simulink model "T37_v65_2015b"  (Simulink 8.6)
settings: Solver=ode45  StartTime=0.0  StopTime=180  FixedStep=0.001  MaxStep=0.1  RelTol=1e-3
values from neighbouring files (symbols this model uses):
  Aero_RP = Aero_RP*[-1 0 0;0 1 0;0 0 -1]    [t37_data.m]
  aileron_limits = [-0.35 0.35]*pi/180    [t37_data.m]
  CD_alpha = 0.3840    (= 0.384)    [t37_data.m]
  CD_beta = [-1.5700	1.2300 ... (first row only)    [t37_data.m]
  CD_flap = 0.0750    (= 0.075)    [t37_data.m]
  CD_zero = [  -1.5700	1.5000 ... (first row only)    [t37_data.m]
  Cl_ail = [0.0000	0.1810 ... (first row only)    [t37_data.m]
  CL_alpha = [-0.2000	-0.6400 ... (first row only)    [t37_data.m]
  CL_alpha_dot = 2.0    (= 2)    [t37_data.m]
  Cl_beta = -0.0944    [t37_data.m]
  CL_elev = 0.5    [t37_data.m]
  CL_flap = 0.3500    (= 0.35)    [t37_data.m]
  CL_ground_effect = [0.0000	1.0610 ... (first row only)    [t37_data.m]
  Cl_p = -0.4420    (= -0.442)    [t37_data.m]
  CL_q = 4.1    [t37_data.m]
  Cl_r = 0.0926    [t37_data.m]
  Cl_rudder = 0.0150    (= 0.015)    [t37_data.m]
  Cm_alpha = -0.7000    (= -0.7)    [t37_data.m]
  Cm_alpha_dot = -6.9500    (= -6.95)    [t37_data.m]
  Cm_elev = [0.0000	-1.1200 ... (first row only)    [t37_data.m]
  Cm_q = -50.0000    (= -50)    [t37_data.m]
  Cm_zero = 0.0250    (= 0.025)    [t37_data.m]
  Cn_beta = 0.1106    [t37_data.m]
  Cn_p = -0.0243    [t37_data.m]
  Cn_r = -0.1390    (= -0.139)    [t37_data.m]
  Cn_rudder = -0.0365    [t37_data.m]
  CY_beta = -0.3460    (= -0.346)    [t37_data.m]
  CY_p = -0.0827    [t37_data.m]
  CY_r = 0.3000    (= 0.3)    [t37_data.m]
  CY_rudder = 0.200    (= 0.2)    [t37_data.m]
  elevator_limits = [-0.35 0.3]*pi/180    [t37_data.m]
  isTrimming = 0    [mytrim.m]    (also in t37_data.m)
  Jxx = 7985*1.3558179    (= 10826.2059315)    [t37_data.m]
  Jxz = 0    [t37_data.m]
  Jyy = 6000*1.3558179    (= 8134.9074)    [t37_data.m]
  Jzz = 11183*1.3558179    (= 15162.1115757)    [t37_data.m]
  M = 4056*0.45359237    (= 1839.77065272)    [t37_data.m]
  Rcg = Rcg*[-1 0 0;0 1 0;0 0 -1]    [t37_data.m]
  Rengine1 = Rengine1*[-1 0 0;0 1 0;0 0 -1]    [t37_data.m]
  Rengine2 = Rengine2*[-1 0 0;0 1 0;0 0 -1]    [t37_data.m]
  rudder_limits = [-0.35 0.35]*pi/180    [t37_data.m]
  Sw = 182*0.09290304    (= 16.90835328)    [t37_data.m]
  thrust_limits = [0 1]    [t37_data.m]
  Tmax = M*10    (= 18397.7065272)    [t37_data.m]
  u0 = [ ... (first row only)    [mytrim.m]    (also in t37_data.m = zeros(4,1))
  x0 = [ ... (first row only)    [mytrim.m]    (also in t37_data.m = zeros(12,1))
undefined symbols (not defined in the file or in its folder): CD_elevator
undefined symbols (not defined in the file): Bw, Cw
(part 2 of 2)

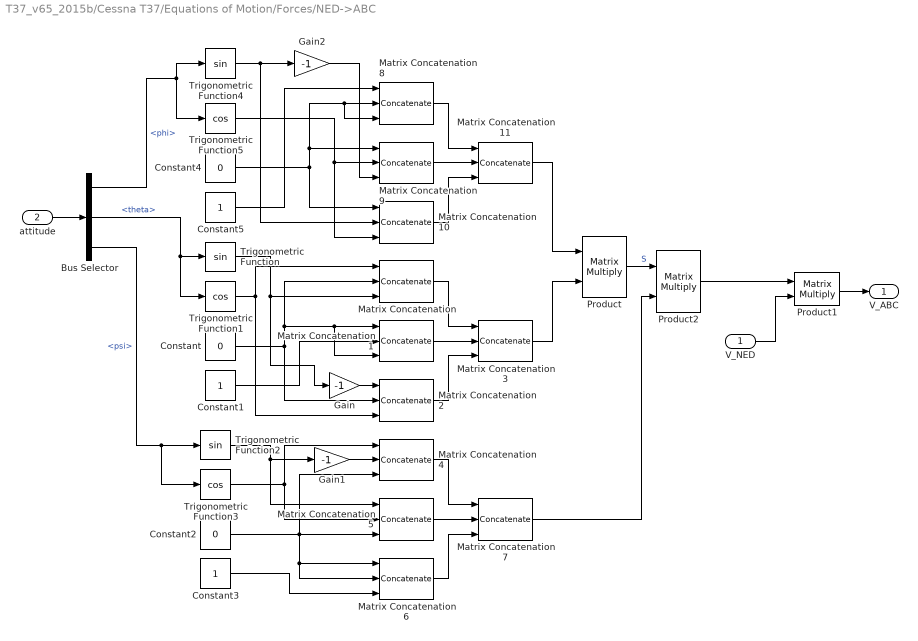
== system T37_v65_2015b/Cessna T37/Equations of Motion/Forces/NED->ABC ==
  V_NED : Inport
  attitude : Inport  Port=2
  Bus Selector : BusSelector  OutputSignals=phi,theta,psi
  Constant : Constant  Value=0
  Constant1 : Constant
  Constant2 : Constant  Value=0
  Constant3 : Constant
  Constant4 : Constant  Value=0
  Constant5 : Constant
  Gain : Gain  Gain=-1  SaturateOnIntegerOverflow=on  OutDataTypeStr=Inherit: Same as input  ParamDataTypeStr=Inherit: Same as input
  Gain1 : Gain  Gain=-1  SaturateOnIntegerOverflow=on  OutDataTypeStr=Inherit: Same as input  ParamDataTypeStr=Inherit: Same as input
  Gain2 : Gain  Gain=-1  SaturateOnIntegerOverflow=on  OutDataTypeStr=Inherit: Same as input  ParamDataTypeStr=Inherit: Same as input
  Matrix Concatenation{,1..2,4..6,8..10} (9 alike) : Concatenate  NumInputs=3  Mode=Multidimensional array
  Matrix Concatenation11 : Concatenate  NumInputs=3  Mode=Multidimensional array  ConcatenateDimension=2
  Matrix Concatenation3 : Concatenate  NumInputs=3  Mode=Multidimensional array  ConcatenateDimension=2
  Matrix Concatenation7 : Concatenate  NumInputs=3  Mode=Multidimensional array  ConcatenateDimension=2
  Product : Product  Multiplication=Matrix(*)  SaturateOnIntegerOverflow=on  OutDataTypeStr=Inherit: Same as first input
  Product1 : Product  Multiplication=Matrix(*)  SaturateOnIntegerOverflow=on  OutDataTypeStr=Inherit: Same as first input
  Product2 : Product  Multiplication=Matrix(*)  SaturateOnIntegerOverflow=on  OutDataTypeStr=Inherit: Same as first input
  Trigonometric Function : Trigonometry
  Trigonometric Function1 : Trigonometry  Operator=cos
  Trigonometric Function2 : Trigonometry
  Trigonometric Function3 : Trigonometry  Operator=cos
  Trigonometric Function4 : Trigonometry
  Trigonometric Function5 : Trigonometry  Operator=cos
  V_ABC : Outport
  wires:
  Trigonometric Function1/1 -> Matrix Concatenation/1, Matrix Concatenation2/3
  Trigonometric Function/1 -> Matrix Concatenation/3, Gain/1
  Constant/1 -> Matrix Concatenation/2, Matrix Concatenation1/1, Matrix Concatenation1/3, Matrix Concatenation2/2
  Constant1/1 -> Matrix Concatenation1/2
  Matrix Concatenation/1 -> Matrix Concatenation3/1
  Matrix Concatenation1/1 -> Matrix Concatenation3/2
  Matrix Concatenation2/1 -> Matrix Concatenation3/3
  Matrix Concatenation4/1 -> Matrix Concatenation7/1
  Matrix Concatenation5/1 -> Matrix Concatenation7/2
  Matrix Concatenation6/1 -> Matrix Concatenation7/3
  Trigonometric Function3/1 -> Matrix Concatenation4/1, Matrix Concatenation5/2
  Trigonometric Function2/1 -> Gain1/1, Matrix Concatenation5/1
  Constant2/1 -> Matrix Concatenation4/3, Matrix Concatenation5/3, Matrix Concatenation6/1, Matrix Concatenation6/2
  Constant3/1 -> Matrix Concatenation6/3
  Product1/1 -> V_ABC/1
  attitude/1 -> Bus Selector/1
  Matrix Concatenation8/1 -> Matrix Concatenation11/1
  Matrix Concatenation9/1 -> Matrix Concatenation11/2
  Matrix Concatenation10/1 -> Matrix Concatenation11/3
  Bus Selector/1 -> Trigonometric Function4/1, Trigonometric Function5/1  "<phi>"
  Constant5/1 -> Matrix Concatenation8/1
  Constant4/1 -> Matrix Concatenation8/2, Matrix Concatenation8/3, Matrix Concatenation9/1, Matrix Concatenation10/1
  Trigonometric Function5/1 -> Matrix Concatenation9/2, Matrix Concatenation10/3
  Trigonometric Function4/1 -> Matrix Concatenation10/2, Gain2/1
  Bus Selector/2 -> Trigonometric Function/1, Trigonometric Function1/1  "<theta>"
  Bus Selector/3 -> Trigonometric Function2/1, Trigonometric Function3/1  "<psi>"
  Matrix Concatenation11/1 -> Product/1
  Matrix Concatenation3/1 -> Product/2
  V_NED/1 -> Product1/2
  Product/1 -> Product2/1  "S"
  Matrix Concatenation7/1 -> Product2/2
  Product2/1 -> Product1/1
  Gain2/1 -> Matrix Concatenation9/3
  Gain/1 -> Matrix Concatenation2/1
  Gain1/1 -> Matrix Concatenation4/2

== system T37_v65_2015b/Cessna T37/Equations of Motion/Forces/Produto Vetorial ==
  V1 : Inport
  V2 : Inport  Port=2
  Mux : Mux  Inputs=2
  Mux1 : Mux  Inputs=3
  i : Fcn  Expr=u(2)*u(6)-u(3)*u(5)
  j : Fcn  Expr=-u(1)*u(6)+u(3)*u(4)
  k : Fcn  Expr=u(1)*u(5)-u(2)*u(4)
  V1 x V2 : Outport
  wires:
  V1/1 -> Mux/1
  V2/1 -> Mux/2
  Mux/1 -> i/1, j/1, k/1
  i/1 -> Mux1/1
  j/1 -> Mux1/2
  k/1 -> Mux1/3
  Mux1/1 -> V1 x V2/1

== system T37_v65_2015b/Cessna T37/Equations of Motion/Forces/Produto Vetorial1 ==
  V1 : Inport
  V2 : Inport  Port=2
  Mux : Mux  Inputs=2
  Mux1 : Mux  Inputs=3
  i : Fcn  Expr=u(2)*u(6)-u(3)*u(5)
  j : Fcn  Expr=-u(1)*u(6)+u(3)*u(4)
  k : Fcn  Expr=u(1)*u(5)-u(2)*u(4)
  V1 x V2 : Outport
  wires:
  V1/1 -> Mux/1
  V2/1 -> Mux/2
  Mux/1 -> i/1, j/1, k/1
  i/1 -> Mux1/1
  j/1 -> Mux1/2
  k/1 -> Mux1/3
  Mux1/1 -> V1 x V2/1

== system T37_v65_2015b/Cessna T37/Equations of Motion/Forces/Produto Vetorial2 ==
  V1 : Inport
  V2 : Inport  Port=2
  Mux : Mux  Inputs=2
  Mux1 : Mux  Inputs=3
  i : Fcn  Expr=u(2)*u(6)-u(3)*u(5)
  j : Fcn  Expr=-u(1)*u(6)+u(3)*u(4)
  k : Fcn  Expr=u(1)*u(5)-u(2)*u(4)
  V1 x V2 : Outport
  wires:
  V1/1 -> Mux/1
  V2/1 -> Mux/2
  Mux/1 -> i/1, j/1, k/1
  i/1 -> Mux1/1
  j/1 -> Mux1/2
  k/1 -> Mux1/3
  Mux1/1 -> V1 x V2/1

== system T37_v65_2015b/Cessna T37/Equations of Motion/Forces/Produto Vetorial3 ==
  V1 : Inport
  V2 : Inport  Port=2
  Mux : Mux  Inputs=2
  Mux1 : Mux  Inputs=3
  i : Fcn  Expr=u(2)*u(6)-u(3)*u(5)
  j : Fcn  Expr=-u(1)*u(6)+u(3)*u(4)
  k : Fcn  Expr=u(1)*u(5)-u(2)*u(4)
  V1 x V2 : Outport
  wires:
  V1/1 -> Mux/1
  V2/1 -> Mux/2
  Mux/1 -> i/1, j/1, k/1
  i/1 -> Mux1/1
  j/1 -> Mux1/2
  k/1 -> Mux1/3
  Mux1/1 -> V1 x V2/1

== system T37_v65_2015b/Cessna T37/Equations of Motion/Moments/Inertia ==
  Constant : Constant  Value=Jxx
  Constant1 : Constant  Value=Jyy
  Constant2 : Constant  Value=Jzz
  Constant3 : Constant  Value=-Jxz
  Constant4 : Constant  Value=0
  Matrix Concatenation10 : Concatenate  NumInputs=3  Mode=Multidimensional array
  Matrix Concatenation11 : Concatenate  NumInputs=3  Mode=Multidimensional array  ConcatenateDimension=2
  Matrix Concatenation8 : Concatenate  NumInputs=3  Mode=Multidimensional array
  Matrix Concatenation9 : Concatenate  NumInputs=3  Mode=Multidimensional array
  J : Outport
  wires:
  Matrix Concatenation8/1 -> Matrix Concatenation11/1
  Matrix Concatenation9/1 -> Matrix Concatenation11/2
  Matrix Concatenation10/1 -> Matrix Concatenation11/3
  Matrix Concatenation11/1 -> J/1
  Constant/1 -> Matrix Concatenation8/1
  Constant4/1 -> Matrix Concatenation8/2, Matrix Concatenation9/1, Matrix Concatenation9/3, Matrix Concatenation10/2
  Constant3/1 -> Matrix Concatenation8/3, Matrix Concatenation10/1
  Constant1/1 -> Matrix Concatenation9/2
  Constant2/1 -> Matrix Concatenation10/3

== system T37_v65_2015b/Cessna T37/Equations of Motion/Moments/Inverse Inertia Matrix ==
  Constant : Constant  Value=Jzz
  Constant1 : Constant  Value=1/Jyy
  Constant2 : Constant  Value=Jxx
  Constant3 : Constant  Value=Jxz
  Constant4 : Constant  Value=0
  Constant5 : Constant  Value=Jxx*Jzz-Jxz^2
  Matrix Concatenation10 : Concatenate  NumInputs=3  Mode=Multidimensional array
  Matrix Concatenation11 : Concatenate  NumInputs=3  Mode=Multidimensional array  ConcatenateDimension=2
  Matrix Concatenation8 : Concatenate  NumInputs=3  Mode=Multidimensional array
  Matrix Concatenation9 : Concatenate  NumInputs=3  Mode=Multidimensional array
  Product : Product  Inputs=*/  SaturateOnIntegerOverflow=on  OutDataTypeStr=Inherit: Same as first input
  Product1 : Product  SaturateOnIntegerOverflow=on  OutDataTypeStr=Inherit: Same as first input
  inv J : Outport
  wires:
  Matrix Concatenation8/1 -> Matrix Concatenation11/1
  Matrix Concatenation9/1 -> Matrix Concatenation11/2
  Matrix Concatenation10/1 -> Matrix Concatenation11/3
  Constant/1 -> Matrix Concatenation8/1
  Constant4/1 -> Matrix Concatenation8/2, Matrix Concatenation9/1, Matrix Concatenation9/3, Matrix Concatenation10/2
  Constant3/1 -> Matrix Concatenation8/3, Matrix Concatenation10/1
  Constant2/1 -> Matrix Concatenation10/3
  Matrix Concatenation11/1 -> Product/1
  Product/1 -> inv J/1
  Constant5/1 -> Product/2, Product1/2
  Constant1/1 -> Product1/1
  Product1/1 -> Matrix Concatenation9/2

== system T37_v65_2015b/Cessna T37/Equations of Motion/Moments/Produto Vetorial1 ==
  V1 : Inport
  V2 : Inport  Port=2
  Mux : Mux  Inputs=2
  Mux1 : Mux  Inputs=3
  i : Fcn  Expr=u(2)*u(6)-u(3)*u(5)
  j : Fcn  Expr=-u(1)*u(6)+u(3)*u(4)
  k : Fcn  Expr=u(1)*u(5)-u(2)*u(4)
  V1 x V2 : Outport
  wires:
  V1/1 -> Mux/1
  V2/1 -> Mux/2
  Mux/1 -> i/1, j/1, k/1
  i/1 -> Mux1/1
  j/1 -> Mux1/2
  k/1 -> Mux1/3
  Mux1/1 -> V1 x V2/1

== system T37_v65_2015b/Cessna T37/Equations of Motion/Moments/Produto Vetorial2 ==
  V1 : Inport
  V2 : Inport  Port=2
  Mux : Mux  Inputs=2
  Mux1 : Mux  Inputs=3
  i : Fcn  Expr=u(2)*u(6)-u(3)*u(5)
  j : Fcn  Expr=-u(1)*u(6)+u(3)*u(4)
  k : Fcn  Expr=u(1)*u(5)-u(2)*u(4)
  V1 x V2 : Outport
  wires:
  V1/1 -> Mux/1
  V2/1 -> Mux/2
  Mux/1 -> i/1, j/1, k/1
  i/1 -> Mux1/1
  j/1 -> Mux1/2
  k/1 -> Mux1/3
  Mux1/1 -> V1 x V2/1

== system T37_v65_2015b/Cessna T37/Equations of Motion/Moments/Produto Vetorial3 ==
  V1 : Inport
  V2 : Inport  Port=2
  Mux : Mux  Inputs=2
  Mux1 : Mux  Inputs=3
  i : Fcn  Expr=u(2)*u(6)-u(3)*u(5)
  j : Fcn  Expr=-u(1)*u(6)+u(3)*u(4)
  k : Fcn  Expr=u(1)*u(5)-u(2)*u(4)
  V1 x V2 : Outport
  wires:
  V1/1 -> Mux/1
  V2/1 -> Mux/2
  Mux/1 -> i/1, j/1, k/1
  i/1 -> Mux1/1
  j/1 -> Mux1/2
  k/1 -> Mux1/3
  Mux1/1 -> V1 x V2/1

== system T37_v65_2015b/Cessna T37/Equations of Motion/Moments/Produto Vetorial4 ==
  V1 : Inport
  V2 : Inport  Port=2
  Mux : Mux  Inputs=2
  Mux1 : Mux  Inputs=3
  i : Fcn  Expr=u(2)*u(6)-u(3)*u(5)
  j : Fcn  Expr=-u(1)*u(6)+u(3)*u(4)
  k : Fcn  Expr=u(1)*u(5)-u(2)*u(4)
  V1 x V2 : Outport
  wires:
  V1/1 -> Mux/1
  V2/1 -> Mux/2
  Mux/1 -> i/1, j/1, k/1
  i/1 -> Mux1/1
  j/1 -> Mux1/2
  k/1 -> Mux1/3
  Mux1/1 -> V1 x V2/1

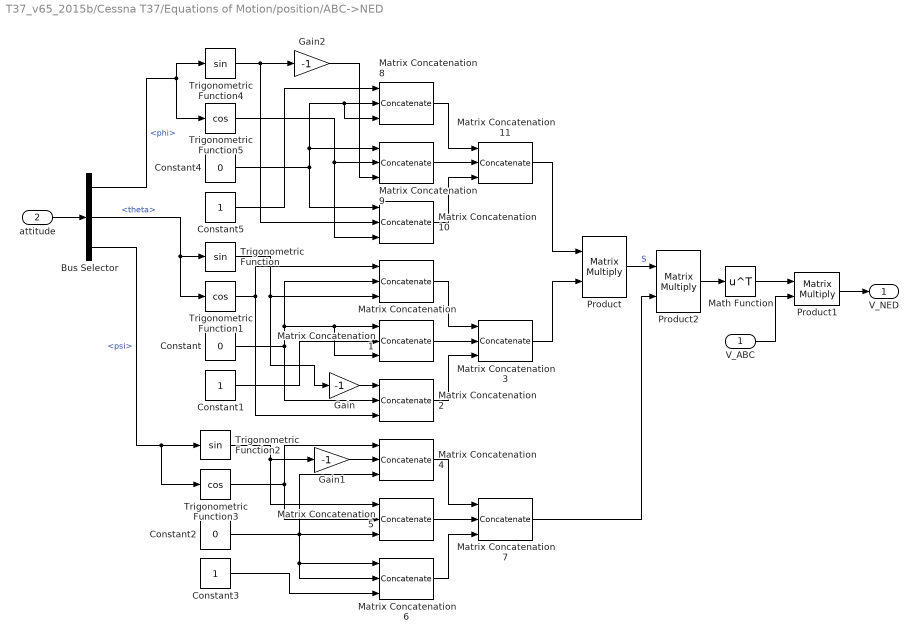
== system T37_v65_2015b/Cessna T37/Equations of Motion/position/ABC->NED ==
  V_ABC : Inport
  attitude : Inport  Port=2
  Bus Selector : BusSelector  OutputSignals=phi,theta,psi
  Constant : Constant  Value=0
  Constant1 : Constant
  Constant2 : Constant  Value=0
  Constant3 : Constant
  Constant4 : Constant  Value=0
  Constant5 : Constant
  Gain : Gain  Gain=-1  SaturateOnIntegerOverflow=on  OutDataTypeStr=Inherit: Same as input  ParamDataTypeStr=Inherit: Same as input
  Gain1 : Gain  Gain=-1  SaturateOnIntegerOverflow=on  OutDataTypeStr=Inherit: Same as input  ParamDataTypeStr=Inherit: Same as input
  Gain2 : Gain  Gain=-1  SaturateOnIntegerOverflow=on  OutDataTypeStr=Inherit: Same as input  ParamDataTypeStr=Inherit: Same as input
  Math Function : Math  Operator=transpose  SaturateOnIntegerOverflow=on
  Matrix Concatenation{,1..2,4..6,8..10} (9 alike) : Concatenate  NumInputs=3  Mode=Multidimensional array
  Matrix Concatenation11 : Concatenate  NumInputs=3  Mode=Multidimensional array  ConcatenateDimension=2
  Matrix Concatenation3 : Concatenate  NumInputs=3  Mode=Multidimensional array  ConcatenateDimension=2
  Matrix Concatenation7 : Concatenate  NumInputs=3  Mode=Multidimensional array  ConcatenateDimension=2
  Product : Product  Multiplication=Matrix(*)  SaturateOnIntegerOverflow=on  OutDataTypeStr=Inherit: Same as first input
  Product1 : Product  Multiplication=Matrix(*)  SaturateOnIntegerOverflow=on  OutDataTypeStr=Inherit: Same as first input
  Product2 : Product  Multiplication=Matrix(*)  SaturateOnIntegerOverflow=on  OutDataTypeStr=Inherit: Same as first input
  Trigonometric Function : Trigonometry
  Trigonometric Function1 : Trigonometry  Operator=cos
  Trigonometric Function2 : Trigonometry
  Trigonometric Function3 : Trigonometry  Operator=cos
  Trigonometric Function4 : Trigonometry
  Trigonometric Function5 : Trigonometry  Operator=cos
  V_NED : Outport
  wires:
  Trigonometric Function1/1 -> Matrix Concatenation/1, Matrix Concatenation2/3
  Trigonometric Function/1 -> Matrix Concatenation/3, Gain/1
  Constant/1 -> Matrix Concatenation/2, Matrix Concatenation1/1, Matrix Concatenation1/3, Matrix Concatenation2/2
  Constant1/1 -> Matrix Concatenation1/2
  Matrix Concatenation/1 -> Matrix Concatenation3/1
  Matrix Concatenation1/1 -> Matrix Concatenation3/2
  Matrix Concatenation2/1 -> Matrix Concatenation3/3
  Matrix Concatenation4/1 -> Matrix Concatenation7/1
  Matrix Concatenation5/1 -> Matrix Concatenation7/2
  Matrix Concatenation6/1 -> Matrix Concatenation7/3
  Trigonometric Function3/1 -> Matrix Concatenation4/1, Matrix Concatenation5/2
  Trigonometric Function2/1 -> Gain1/1, Matrix Concatenation5/1
  Constant2/1 -> Matrix Concatenation4/3, Matrix Concatenation5/3, Matrix Concatenation6/1, Matrix Concatenation6/2
  Constant3/1 -> Matrix Concatenation6/3
  Product1/1 -> V_NED/1
  attitude/1 -> Bus Selector/1
  Matrix Concatenation8/1 -> Matrix Concatenation11/1
  Matrix Concatenation9/1 -> Matrix Concatenation11/2
  Matrix Concatenation10/1 -> Matrix Concatenation11/3
  Bus Selector/1 -> Trigonometric Function4/1, Trigonometric Function5/1  "<phi>"
  Constant5/1 -> Matrix Concatenation8/1
  Constant4/1 -> Matrix Concatenation8/2, Matrix Concatenation8/3, Matrix Concatenation9/1, Matrix Concatenation10/1
  Trigonometric Function5/1 -> Matrix Concatenation9/2, Matrix Concatenation10/3
  Trigonometric Function4/1 -> Matrix Concatenation10/2, Gain2/1
  Bus Selector/2 -> Trigonometric Function/1, Trigonometric Function1/1  "<theta>"
  Bus Selector/3 -> Trigonometric Function2/1, Trigonometric Function3/1  "<psi>"
  Matrix Concatenation11/1 -> Product/1
  Matrix Concatenation3/1 -> Product/2
  V_ABC/1 -> Product1/2
  Product/1 -> Product2/1  "S"
  Matrix Concatenation7/1 -> Product2/2
  Gain2/1 -> Matrix Concatenation9/3
  Gain/1 -> Matrix Concatenation2/1
  Gain1/1 -> Matrix Concatenation4/2
  Product2/1 -> Math Function/1
  Math Function/1 -> Product1/1
